simulink model "FinalRobot"  (R2021b)
settings: Solver=ode23t  StartTime=0.0  StopTime=120  MaxStep=3e-3  RelTol=1e-3
undefined symbols (not defined in the file): Amor1, Amor2, Amor3, Amor4, Amor5, B_Verin1, B_Verin2, B_Verin3, B_Verin4, B_Verin5, H_Verin1, H_Verin2, H_Verin3, H_Verin4, H_Verin5, k, K, Middle_Sensing, Sensing_1, Sensing_2, Wall_1, Wall_10, Wall_11, Wall_2, Wall_3, Wall_4, Wall_5, Wall_6, Wall_7, Wall_8, Wall_9, X, Y, Z
libraries: sm_lib x237, nesl_utility x60
(part 2 of 8)

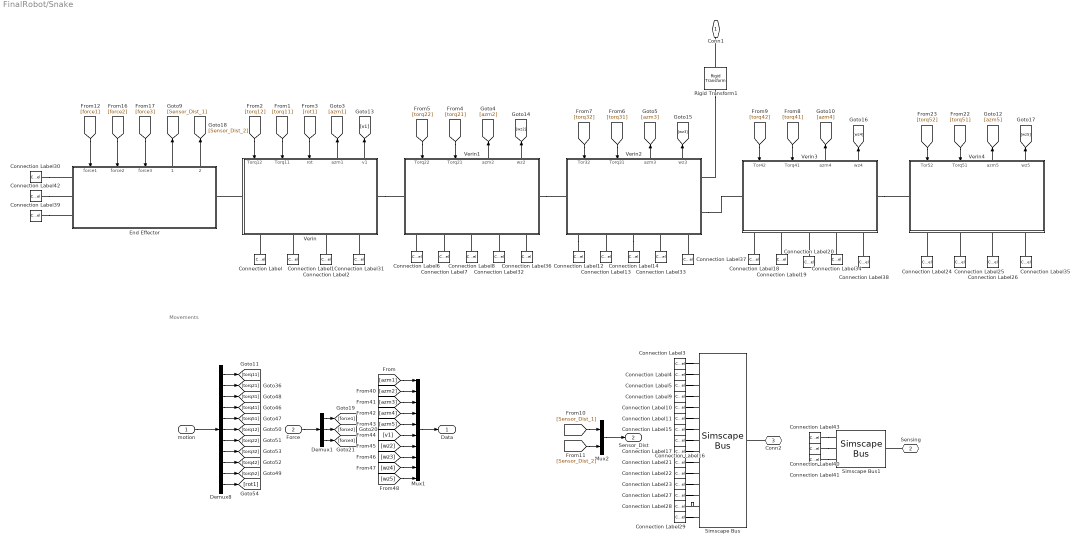
== system FinalRobot/Snake ==
  note: Movements
  motion : Inport
  Force : Inport  Port=2
  Connection Label : ConnectionLabel
  Connection Label1 : ConnectionLabel  Label=Label2
  Connection Label10 : ConnectionLabel  Label=Label5
  Connection Label11 : ConnectionLabel  Label=Label6
  Connection Label12 : ConnectionLabel  Label=Label7
  Connection Label13 : ConnectionLabel  Label=Label8
  Connection Label14 : ConnectionLabel  Label=Label9
  Connection Label15 : ConnectionLabel  Label=Label7
  Connection Label16 : ConnectionLabel  Label=Label8
  Connection Label17 : ConnectionLabel  Label=Label9
  Connection Label18 : ConnectionLabel  Label=Label10
  Connection Label19 : ConnectionLabel  Label=Label11
  Connection Label2 : ConnectionLabel  Label=Label3
  Connection Label20 : ConnectionLabel  Label=Label12
  Connection Label21 : ConnectionLabel  Label=Label10
  Connection Label22 : ConnectionLabel  Label=Label11
  Connection Label23 : ConnectionLabel  Label=Label12
  Connection Label24 : ConnectionLabel  Label=Label13
  Connection Label25 : ConnectionLabel  Label=Label14
  Connection Label26 : ConnectionLabel  Label=Label15
  Connection Label27 : ConnectionLabel  Label=Label13
  Connection Label28 : ConnectionLabel  Label=Label14
  Connection Label29 : ConnectionLabel  Label=Label15
  Connection Label3 : ConnectionLabel
  Connection Label30 : ConnectionLabel  Label=Label16
  Connection Label31 : ConnectionLabel  Label=Ref1
  Connection Label32 : ConnectionLabel  Label=Ref1
  Connection Label33 : ConnectionLabel  Label=Ref2
  Connection Label34 : ConnectionLabel  Label=Ref3
  Connection Label35 : ConnectionLabel  Label=Ref4
  Connection Label36 : ConnectionLabel  Label=Ref2
  Connection Label37 : ConnectionLabel  Label=Ref3
  Connection Label38 : ConnectionLabel  Label=Ref4
  Connection Label39 : ConnectionLabel  Label=Label17
  Connection Label4 : ConnectionLabel  Label=Label2
  Connection Label40 : ConnectionLabel  Label=Label16
  Connection Label41 : ConnectionLabel  Label=Label17
  Connection Label42 : ConnectionLabel  Label=Label18
  Connection Label43 : ConnectionLabel  Label=Label18
  Connection Label5 : ConnectionLabel  Label=Label3
  Connection Label6 : ConnectionLabel  Label=Label4
  Connection Label7 : ConnectionLabel  Label=Label5
  Connection Label8 : ConnectionLabel  Label=Label6
  Connection Label9 : ConnectionLabel  Label=Label4
  Demux1 : Demux  Outputs=3
  Demux8 : Demux  Outputs=11
  End Effector : Subsystem
      settings: PortSchema="{\"entries\":[{\"content\":{\"sides\":[{\"content\":{\"connectorIds\":[\"LConn1\",\"LConn2\",\"LConn3\"]},\"type\":\"ConnectorPlacement.EquallySpacedRectSide\",\"uuid\":\"5cdd056e-886a-4e79-8899-044af396038d\"},{\"content\":{\"connectorIds\":[\"RConn1\"],\"side\":\"RIGHT\"},\"type\":\"ConnectorPlacement.EquallySpacedRectSide\",\"uuid\":\"cf985096-d37a-46e5-b464-4af5c863f88b\"},{\"content\":{\"connectorIds\":[\"In1\",\"In2\",\"In3\",\"Out1\",\"Out2\"],\"side\":\"TOP\"},\"type\":\"ConnectorPlacement.EquallySpacedRectSide\",\"uuid\":\"be1169e8-83ff-4042-b398-0e1dc3f716bc\"}]},\"type\":\"ConnectorPlacement.EquallySpacedConnector\",\"uuid\":\"d39d92c9-4302-400d-962a-d4b186813480\"}],\"packageUris\":[\"http://schema.mathworks.com/mf0/Connector/R2020b\"],\"version\":\"1.0\"}"
      mask Display: image('$imagefile'); % Use "Edit Image" on toolstrip to change.
  Mux1 : Mux  Inputs=10
  Mux2 : Mux  Inputs=2
  Rigid Transform1 : sm_lib/Frames and Transforms/Rigid Transform  TranslationMethod=Cartesian  TranslationStandardOffset=0  TranslationLengthUnit=m  TranslationStandardAxis=+Z  TranslationCartesianOffset=[-0.1 -0.2 0.1]  TranslationROffset=0  TranslationROffsetUnits=m  TranslationZOffset=0  TranslationZOffsetUnits=m  TranslationThetaOffset=0  TranslationThetaOffsetUnits=deg  RotationMethod=StandardAxis  RotationAngleUnits=deg  RotationStandardAxis=+Z  RotationAngle=30  RotationArbitraryAxis=[0 0 1]  FollAlignAxisA=+X  BaseAlignAxisA=+Y  FollAlignAxisB=+Y  BaseAlignAxisB=+Z  RotationSequenceAxes=FollowerAxes  RotationSequence=XYX  RotationSequenceAngles=[0 0 0]  RotationSequenceAnglesUnits=deg  RotationMatrix=[1 0 0; 0 1 0; 0 0 1]
  Simscape Bus : SimscapeBus  HierarchyStrings=Amor1;H_Verin1;B_Verin1;Amor2;H_Verin2;B_Verin2;Amor3;H_Verin3;B_Verin3;Amor4;H_Verin4;B_Verin4;Amor5;H_Verin5;B_Verin5
  Simscape Bus1 : SimscapeBus  HierarchyStrings=Middle_Sensing;Sensing_1;Sensing_2
  Verin : Subsystem
      settings: PortSchema="{\"entries\":[{\"content\":{\"sides\":[{\"content\":{\"connectorIds\":[\"LConn1\"]},\"type\":\"ConnectorPlacement.EquallySpacedRectSide\",\"uuid\":\"c3246ee3-eb2d-4c48-a7f8-29eef62ed6cd\"},{\"content\":{\"connectorIds\":[\"RConn1\"],\"side\":\"RIGHT\"},\"type\":\"ConnectorPlacement.EquallySpacedRectSide\",\"uuid\":\"dd74c587-cb0d-4684-823f-ccc260fba800\"},{\"content\":{\"connectorIds\":[\"In1\",\"In2\",\"In3\",\"Out1\",\"Out2\"],\"side\":\"TOP\"},\"type\":\"ConnectorPlacement.EquallySpacedRectSide\",\"uuid\":\"65ea7381-0dcf-4a70-96d8-66f9da1f3035\"},{\"content\":{\"connectorIds\":[\"RConn2\",\"RConn3\",\"RConn4\",\"RConn5\"],\"side\":\"BOTTOM\"},\"type\":\"ConnectorPlacement.EquallySpacedRectSide\",\"uuid\":\"fb9c5bb7-17a2-4c30-b9f8-fa15cd56ac19\"}]},\"type\":\"ConnectorPlacement.EquallySpacedConnector\",\"uuid\":\"772b1dde-44da-42b0-bd8c-81ff8dd9042a\"}],\"packageUris\":[\"http://schema.mathworks.com/mf0/Connector/R2020b\"],\"version\":\"1.0\"}"
      mask Display: image('$imagefile'); % Use "Edit Image" on toolstrip to change.
  Verin1 : Subsystem
      settings: PortSchema="{\"entries\":[{\"content\":{\"sides\":[{\"content\":{\"connectorIds\":[\"LConn1\"]},\"type\":\"ConnectorPlacement.EquallySpacedRectSide\",\"uuid\":\"c3246ee3-eb2d-4c48-a7f8-29eef62ed6cd\"},{\"content\":{\"connectorIds\":[\"RConn1\"],\"side\":\"RIGHT\"},\"type\":\"ConnectorPlacement.EquallySpacedRectSide\",\"uuid\":\"dd74c587-cb0d-4684-823f-ccc260fba800\"},{\"content\":{\"connectorIds\":[\"In1\",\"In2\",\"Out1\",\"Out2\"],\"side\":\"TOP\"},\"type\":\"ConnectorPlacement.EquallySpacedRectSide\",\"uuid\":\"65ea7381-0dcf-4a70-96d8-66f9da1f3035\"},{\"content\":{\"connectorIds\":[\"RConn2\",\"RConn3\",\"RConn4\",\"RConn5\",\"RConn6\"],\"side\":\"BOTTOM\"},\"type\":\"ConnectorPlacement.EquallySpacedRectSide\",\"uuid\":\"fb9c5bb7-17a2-4c30-b9f8-fa15cd56ac19\"}]},\"type\":\"ConnectorPlacement.EquallySpacedConnector\",\"uuid\":\"772b1dde-44da-42b0-bd8c-81ff8dd9042a\"}],\"packageUris\":[\"http://schema.mathworks.com/mf0/Connector/R2020b\"],\"version\":\"1.0\"}"
      mask Display: image('$imagefile'); % Use "Edit Image" on toolstrip to change.
  Verin2 : Subsystem
      settings: PortSchema="{\"entries\":[{\"content\":{\"sides\":[{\"content\":{\"connectorIds\":[\"LConn1\"]},\"type\":\"ConnectorPlacement.EquallySpacedRectSide\",\"uuid\":\"c3246ee3-eb2d-4c48-a7f8-29eef62ed6cd\"},{\"content\":{\"connectorIds\":[\"RConn1\",\"RConn2\"],\"side\":\"RIGHT\"},\"type\":\"ConnectorPlacement.EquallySpacedRectSide\",\"uuid\":\"dd74c587-cb0d-4684-823f-ccc260fba800\"},{\"content\":{\"connectorIds\":[\"In1\",\"In2\",\"Out1\",\"Out2\"],\"side\":\"TOP\"},\"type\":\"ConnectorPlacement.EquallySpacedRectSide\",\"uuid\":\"65ea7381-0dcf-4a70-96d8-66f9da1f3035\"},{\"content\":{\"connectorIds\":[\"RConn3\",\"RConn4\",\"RConn5\",\"RConn6\",\"RConn7\"],\"side\":\"BOTTOM\"},\"type\":\"ConnectorPlacement.EquallySpacedRectSide\",\"uuid\":\"fb9c5bb7-17a2-4c30-b9f8-fa15cd56ac19\"}]},\"type\":\"ConnectorPlacement.EquallySpacedConnector\",\"uuid\":\"772b1dde-44da-42b0-bd8c-81ff8dd9042a\"}],\"packageUris\":[\"http://schema.mathworks.com/mf0/Connector/R2020b\"],\"version\":\"1.0\"}"
      mask Display: image('$imagefile'); % Use "Edit Image" on toolstrip to change.
  Verin3 : Subsystem
      settings: PortSchema="{\"entries\":[{\"content\":{\"sides\":[{\"content\":{\"connectorIds\":[\"LConn1\"]},\"type\":\"ConnectorPlacement.EquallySpacedRectSide\",\"uuid\":\"c3246ee3-eb2d-4c48-a7f8-29eef62ed6cd\"},{\"content\":{\"connectorIds\":[\"RConn1\"],\"side\":\"RIGHT\"},\"type\":\"ConnectorPlacement.EquallySpacedRectSide\",\"uuid\":\"dd74c587-cb0d-4684-823f-ccc260fba800\"},{\"content\":{\"connectorIds\":[\"In1\",\"In2\",\"Out1\",\"Out2\"],\"side\":\"TOP\"},\"type\":\"ConnectorPlacement.EquallySpacedRectSide\",\"uuid\":\"65ea7381-0dcf-4a70-96d8-66f9da1f3035\"},{\"content\":{\"connectorIds\":[\"RConn2\",\"RConn3\",\"RConn4\",\"RConn5\",\"RConn6\"],\"side\":\"BOTTOM\"},\"type\":\"ConnectorPlacement.EquallySpacedRectSide\",\"uuid\":\"fb9c5bb7-17a2-4c30-b9f8-fa15cd56ac19\"}]},\"type\":\"ConnectorPlacement.EquallySpacedConnector\",\"uuid\":\"772b1dde-44da-42b0-bd8c-81ff8dd9042a\"}],\"packageUris\":[\"http://schema.mathworks.com/mf0/Connector/R2020b\"],\"version\":\"1.0\"}"
      mask Display: image('$imagefile'); % Use "Edit Image" on toolstrip to change.
  Verin4 : Subsystem
      settings: PortSchema="{\"entries\":[{\"content\":{\"sides\":[{\"content\":{\"connectorIds\":[\"LConn1\"]},\"type\":\"ConnectorPlacement.EquallySpacedRectSide\",\"uuid\":\"c3246ee3-eb2d-4c48-a7f8-29eef62ed6cd\"},{\"content\":{\"connectorIds\":[],\"side\":\"RIGHT\"},\"type\":\"ConnectorPlacement.EquallySpacedRectSide\",\"uuid\":\"dd74c587-cb0d-4684-823f-ccc260fba800\"},{\"content\":{\"connectorIds\":[\"In1\",\"In2\",\"Out1\",\"Out2\"],\"side\":\"TOP\"},\"type\":\"ConnectorPlacement.EquallySpacedRectSide\",\"uuid\":\"65ea7381-0dcf-4a70-96d8-66f9da1f3035\"},{\"content\":{\"connectorIds\":[\"RConn1\",\"RConn2\",\"RConn3\",\"RConn4\"],\"side\":\"BOTTOM\"},\"type\":\"ConnectorPlacement.EquallySpacedRectSide\",\"uuid\":\"fb9c5bb7-17a2-4c30-b9f8-fa15cd56ac19\"}]},\"type\":\"ConnectorPlacement.EquallySpacedConnector\",\"uuid\":\"772b1dde-44da-42b0-bd8c-81ff8dd9042a\"}],\"packageUris\":[\"http://schema.mathworks.com/mf0/Connector/R2020b\"],\"version\":\"1.0\"}"
      mask Display: image('$imagefile'); % Use "Edit Image" on toolstrip to change.
  Conn1 : PMIOPort  Side=Left
  Sensing : PMIOPort  Port=2  Side=Right
  Conn2 : PMIOPort  Port=3  Side=Right
  Data : Outport
  Sensor_Dist : Outport  Port=2
  wires:
  [torq41] -> Verin3/2(Torq41)
  [torq22] -> Verin1/1(Torq22)
  [torq52] -> Verin4/1(Tor52)
  Demux8/2 -> [torq21]
  Demux8/6 -> [torq12]
  Demux8/11 -> [rot1]
  [torq11] -> Verin/2(Torq11)
  [rot1] -> Verin/3(rot)
  [torq21] -> Verin1/2(Torq21)
  [torq51] -> Verin4/2(Torq51)
  [torq42] -> Verin3/1(Tor42)
  Demux8/9 -> [torq42]
  Demux8/7 -> [torq22]
  [torq32] -> Verin2/1(Tor32)
  Demux8/3 -> [torq31]
  Demux8/4 -> [torq41]
  [torq31] -> Verin2/2(Torq31)
  [torq12] -> Verin/1(Torq12)
  Demux8/10 -> [torq52]
  Demux8/5 -> [torq51]
  Demux8/1 -> [torq11]
  Demux8/8 -> [torq32]
  motion/1 -> Demux8/1
  Mux1/1 -> Data/1
  [azm1] -> Mux1/1
  Verin/1(azm1) -> [azm1]
  Verin1/1(azm2) -> [azm2]
  Verin2/1(azm3) -> [azm3]
  Verin3/1(azm4) -> [azm4]
  Verin4/1(azm5) -> [azm5]
  [azm2] -> Mux1/2
  [azm3] -> Mux1/3
  [azm4] -> Mux1/4
  [azm5] -> Mux1/5
  Verin/2(v1) -> [v1]
  Verin1/2(wz2) -> [wz2]
  Verin2/2(wz3) -> [wz3]
  Verin3/2(wz4) -> [wz4]
  Verin4/2(wz5) -> [wz5]
  [wz3] -> Mux1/8
  [wz2] -> Mux1/7
  [v1] -> Mux1/6
  [wz4] -> Mux1/9
  [wz5] -> Mux1/10
  End Effector/1(Sensor_Dist_1) -> [Sensor_Dist_1]
  End Effector/2(Sensor_Dist_2) -> [Sensor_Dist_2]
  [Sensor_Dist_1] -> Mux2/1
  [Sensor_Dist_2] -> Mux2/2
  Mux2/1 -> Sensor_Dist/1
  Force/1 -> Demux1/1
  Demux1/1 -> [force1]
  Demux1/2 -> [force2]
  Demux1/3 -> [force3]
  [force2] -> End Effector/2(force2)
  [force1] -> End Effector/1(force1)
  [force3] -> End Effector/3(force3)
  connections:
  Verin2/RConn2 -- Verin3/LConn1
  Verin3/RConn1 -- Verin4/LConn1
  Verin1/RConn1 -- Verin2/LConn1
  Rigid Transform1/LConn1 -- Conn1/RConn1
  Conn2/RConn1 -- Simscape Bus/RConn1
  Connection Label/LConn1 -- Verin/RConn2
  Connection Label1/LConn1 -- Verin/RConn3
  Connection Label2/LConn1 -- Verin/RConn4
  Connection Label5/LConn1 -- Simscape Bus/LConn3
  Connection Label3/LConn1 -- Simscape Bus/LConn1
  Connection Label4/LConn1 -- Simscape Bus/LConn2
  Connection Label6/LConn1 -- Verin1/RConn2
  Connection Label7/LConn1 -- Verin1/RConn3
  Connection Label8/LConn1 -- Verin1/RConn4
  Connection Label9/LConn1 -- Simscape Bus/LConn4
  Connection Label10/LConn1 -- Simscape Bus/LConn5
  Connection Label11/LConn1 -- Simscape Bus/LConn6
  Verin2/RConn5 -- Connection Label14/LConn1
  Connection Label13/LConn1 -- Verin2/RConn4
  Verin2/RConn3 -- Connection Label12/LConn1
  Connection Label19/LConn1 -- Verin3/RConn3
  Connection Label18/LConn1 -- Verin3/RConn2
  Connection Label20/LConn1 -- Verin3/RConn4
  Connection Label23/LConn1 -- Simscape Bus/LConn12
  Connection Label21/LConn1 -- Simscape Bus/LConn10
  Connection Label22/LConn1 -- Simscape Bus/LConn11
  Connection Label15/LConn1 -- Simscape Bus/LConn7
  Connection Label16/LConn1 -- Simscape Bus/LConn8
  Connection Label17/LConn1 -- Simscape Bus/LConn9
  Connection Label24/LConn1 -- Verin4/RConn1
  Connection Label25/LConn1 -- Verin4/RConn2
  Connection Label26/LConn1 -- Verin4/RConn3
  Connection Label27/LConn1 -- Simscape Bus/LConn13
  Connection Label29/LConn1 -- Simscape Bus/LConn15
  Simscape Bus/LConn14 -- Connection Label28/LConn1
  Connection Label31/LConn1 -- Verin/RConn5
  Connection Label32/LConn1 -- Verin1/RConn5
  Connection Label33/LConn1 -- Verin2/RConn6
  Connection Label34/LConn1 -- Verin3/RConn5
  Connection Label35/LConn1 -- Verin4/RConn4
  Connection Label36/LConn1 -- Verin1/RConn6
  Connection Label37/LConn1 -- Verin2/RConn7
  Connection Label38/LConn1 -- Verin3/RConn6
  Rigid Transform1/RConn1 -- Verin2/RConn1
  Sensing/RConn1 -- Simscape Bus1/RConn1
  Connection Label41/LConn1 -- Simscape Bus1/LConn3
  Connection Label40/LConn1 -- Simscape Bus1/LConn2
  Connection Label43/LConn1 -- Simscape Bus1/LConn1
  Connection Label30/LConn1 -- End Effector/LConn1
  Connection Label42/LConn1 -- End Effector/LConn2
  Verin/LConn1 -- End Effector/RConn1
  Connection Label39/LConn1 -- End Effector/LConn3
  Verin/RConn1 -- Verin1/LConn1

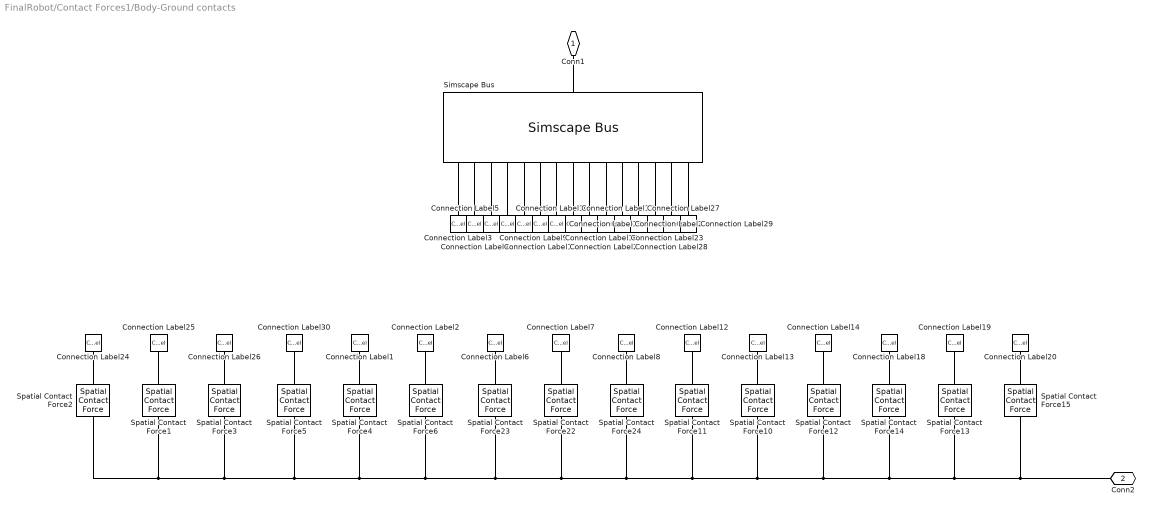
== system FinalRobot/Contact Forces1/Body-Ground contacts ==
  Connection Label1 : ConnectionLabel  Label=Label5
  Connection Label10 : ConnectionLabel  Label=Label5
  Connection Label11 : ConnectionLabel  Label=Label6
  Connection Label12 : ConnectionLabel  Label=Label10
  Connection Label13 : ConnectionLabel  Label=Label11
  Connection Label14 : ConnectionLabel  Label=Label12
  Connection Label15 : ConnectionLabel  Label=Label7
  Connection Label16 : ConnectionLabel  Label=Label8
  Connection Label17 : ConnectionLabel  Label=Label9
  Connection Label18 : ConnectionLabel  Label=Label13
  Connection Label19 : ConnectionLabel  Label=Label14
  Connection Label2 : ConnectionLabel  Label=Label6
  Connection Label20 : ConnectionLabel  Label=Label15
  Connection Label21 : ConnectionLabel  Label=Label10
  Connection Label22 : ConnectionLabel  Label=Label11
  Connection Label23 : ConnectionLabel  Label=Label12
  Connection Label24 : ConnectionLabel
  Connection Label25 : ConnectionLabel  Label=Label2
  Connection Label26 : ConnectionLabel  Label=Label3
  Connection Label27 : ConnectionLabel  Label=Label13
  Connection Label28 : ConnectionLabel  Label=Label14
  Connection Label29 : ConnectionLabel  Label=Label15
  Connection Label3 : ConnectionLabel
  Connection Label30 : ConnectionLabel  Label=Label4
  Connection Label4 : ConnectionLabel  Label=Label2
  Connection Label5 : ConnectionLabel  Label=Label3
  Connection Label6 : ConnectionLabel  Label=Label7
  Connection Label7 : ConnectionLabel  Label=Label8
  Connection Label8 : ConnectionLabel  Label=Label9
  Connection Label9 : ConnectionLabel  Label=Label4
  Simscape Bus : SimscapeBus  HierarchyStrings=Amor1;H_Verin1;B_Verin1;Amor2;H_Verin2;B_Verin2;Amor3;H_Verin3;B_Verin3;Amor4;H_Verin4;B_Verin4;Amor5;H_Verin5;B_Verin5
  Spatial Contact Force{1,3..4,6,10,12..13,15,22,24} (10 alike) : sm_lib/Forces and Torques/Spatial Contact Force  CoefficientOfDynamicFriction=Dynamic_Friction_Verin  CoefficientOfStaticFriction=Static_Friction_Verin  SenseContactBaseRotation=off  SenseContactBaseTranslation=off  NormalDamping=1e3  NormalDampingUnits=N/(m/s)  SenseContactFollowerRotation=off  SenseContactFollowerTranslation=off  SenseContactSignal=off  NormalStiffness=1e6  NormalStiffnessUnits=N/m  FrictionalCriticalVelocity=1e-3  FrictionalCriticalVelocityUnits=m/s  ZeroCrossDetectContactStartAndEnd=off  FrictionType=SmoothStickSlip  SenseFrictionalForceMagnitude=off  SenseNormalForceMagnitude=off  NormalForceType=SmoothSpringDamper  SenseNormalVelocity=off  SenseSeparationDistance=off  SenseTangentialVelocity=off  SenseTangentialVelocityMagnitude=off  NormalTransitionRegionWidth=1e-4  NormalTransitionRegionWidthUnits=m
  Spatial Contact Force{2,5,11,14,23} (5 alike) : sm_lib/Forces and Torques/Spatial Contact Force  CoefficientOfDynamicFriction=Dynamic_Friction_Amor  CoefficientOfStaticFriction=Static_Friction_Amor  SenseContactBaseRotation=off  SenseContactBaseTranslation=off  NormalDamping=1e3  NormalDampingUnits=N/(m/s)  SenseContactFollowerRotation=off  SenseContactFollowerTranslation=off  SenseContactSignal=off  NormalStiffness=1e6  NormalStiffnessUnits=N/m  FrictionalCriticalVelocity=1e-3  FrictionalCriticalVelocityUnits=m/s  ZeroCrossDetectContactStartAndEnd=off  FrictionType=SmoothStickSlip  SenseFrictionalForceMagnitude=off  SenseNormalForceMagnitude=off  NormalForceType=SmoothSpringDamper  SenseNormalVelocity=off  SenseSeparationDistance=off  SenseTangentialVelocity=off  SenseTangentialVelocityMagnitude=off  NormalTransitionRegionWidth=1e-4  NormalTransitionRegionWidthUnits=m
  Conn1 : PMIOPort  Side=Left
  Conn2 : PMIOPort  Port=2  Side=Right
  connections:
  Connection Label15/LConn1 -- Simscape Bus/LConn7
  Spatial Contact Force2/LConn1 -- Spatial Contact Force1/LConn1 -- Spatial Contact Force3/LConn1 -- Spatial Contact Force5/LConn1 -- Spatial Contact Force4/LConn1 -- Spatial Contact Force6/LConn1 -- Spatial Contact Force23/LConn1 -- Spatial Contact Force22/LConn1 -- Spatial Contact Force24/LConn1 -- Spatial Contact Force11/LConn1 -- Spatial Contact Force10/LConn1 -- Spatial Contact Force12/LConn1 -- Conn2/RConn1 -- Spatial Contact Force15/LConn1 -- Spatial Contact Force13/LConn1 -- Spatial Contact Force14/LConn1
  Connection Label26/LConn1 -- Spatial Contact Force3/RConn1
  Connection Label30/LConn1 -- Spatial Contact Force5/RConn1
  Connection Label24/LConn1 -- Spatial Contact Force2/RConn1
  Connection Label27/LConn1 -- Simscape Bus/LConn13
  Connection Label29/LConn1 -- Simscape Bus/LConn15
  Connection Label18/LConn1 -- Spatial Contact Force14/RConn1
  Connection Label14/LConn1 -- Spatial Contact Force12/RConn1
  Connection Label20/LConn1 -- Spatial Contact Force15/RConn1
  Connection Label11/LConn1 -- Simscape Bus/LConn6
  Connection Label1/LConn1 -- Spatial Contact Force4/RConn1
  Connection Label8/LConn1 -- Spatial Contact Force24/RConn1
  Connection Label13/LConn1 -- Spatial Contact Force10/RConn1
  Simscape Bus/LConn14 -- Connection Label28/LConn1
  Connection Label25/LConn1 -- Spatial Contact Force1/RConn1
  Connection Label7/LConn1 -- Spatial Contact Force22/RConn1
  Connection Label10/LConn1 -- Simscape Bus/LConn5
  Connection Label16/LConn1 -- Simscape Bus/LConn8
  Connection Label22/LConn1 -- Simscape Bus/LConn11
  Connection Label3/LConn1 -- Simscape Bus/LConn1
  Connection Label17/LConn1 -- Simscape Bus/LConn9
  Connection Label23/LConn1 -- Simscape Bus/LConn12
  Connection Label6/LConn1 -- Spatial Contact Force23/RConn1
  Connection Label4/LConn1 -- Simscape Bus/LConn2
  Connection Label5/LConn1 -- Simscape Bus/LConn3
  Connection Label2/LConn1 -- Spatial Contact Force6/RConn1
  Connection Label12/LConn1 -- Spatial Contact Force11/RConn1
  Connection Label19/LConn1 -- Spatial Contact Force13/RConn1
  Connection Label9/LConn1 -- Simscape Bus/LConn4
  Connection Label21/LConn1 -- Simscape Bus/LConn10
  Conn1/RConn1 -- Simscape Bus/RConn1

== system FinalRobot/Contact Forces1/Subsystem3 ==
  Simscape Bus1 : SimscapeBus  HierarchyStrings=Middle_Sensing;Sensing_1;Sensing_2
  Simscape Bus2 : SimscapeBus  HierarchyStrings=Wall_1;Wall_2;Wall_3;Wall_4;Wall_5;Wall_6;Wall_7;Wall_8;Wall_9;Wall_10;Wall_11
  Subsystem : Subsystem
      settings: PortSchema="{\"entries\":[{\"content\":{\"sides\":[{\"content\":{\"connectorIds\":[]},\"type\":\"ConnectorPlacement.EquallySpacedRectSide\",\"uuid\":\"68d41a2c-cf4f-4266-9bb2-d19176523fa8\"},{\"content\":{\"connectorIds\":[],\"side\":\"RIGHT\"},\"type\":\"ConnectorPlacement.EquallySpacedRectSide\",\"uuid\":\"fed068d2-51f7-41d7-8fa2-5f11aa30b23c\"},{\"content\":{\"connectorIds\":[\"LConn1\",\"Out1\"],\"side\":\"TOP\"},\"type\":\"ConnectorPlacement.EquallySpacedRectSide\",\"uuid\":\"b5637d28-03b4-4ccb-b57f-dccf0e87748a\"},{\"content\":{\"connectorIds\":[\"RConn1\",\"RConn2\",\"RConn3\",\"RConn4\",\"RConn5\",\"RConn6\",\"RConn7\",\"RConn8\",\"RConn9\",\"RConn10\",\"RConn11\"],\"side\":\"BOTTOM\"},\"type\":\"ConnectorPlacement.EquallySpacedRectSide\",\"uuid\":\"554c0383-4a72-43a1-a6a1-ce5953181375\"}]},\"type\":\"ConnectorPlacement.EquallySpacedConnector\",\"uuid\":\"ce1fbdf9-62dc-494f-9c60-f0c11efaa8b9\"}],\"packageUris\":[\"http://schema.mathworks.com/mf0/Connector/R2020b\"],\"version\":\"1.0\"}"
  Subsystem1 : Subsystem
      settings: PortSchema="{\"entries\":[{\"content\":{\"sides\":[{\"content\":{\"connectorIds\":[]},\"type\":\"ConnectorPlacement.EquallySpacedRectSide\",\"uuid\":\"68d41a2c-cf4f-4266-9bb2-d19176523fa8\"},{\"content\":{\"connectorIds\":[],\"side\":\"RIGHT\"},\"type\":\"ConnectorPlacement.EquallySpacedRectSide\",\"uuid\":\"fed068d2-51f7-41d7-8fa2-5f11aa30b23c\"},{\"content\":{\"connectorIds\":[\"LConn1\",\"Out1\"],\"side\":\"TOP\"},\"type\":\"ConnectorPlacement.EquallySpacedRectSide\",\"uuid\":\"b5637d28-03b4-4ccb-b57f-dccf0e87748a\"},{\"content\":{\"connectorIds\":[\"RConn1\",\"RConn2\",\"RConn3\",\"RConn4\",\"RConn5\",\"RConn6\",\"RConn7\",\"RConn8\",\"RConn9\",\"RConn10\",\"RConn11\"],\"side\":\"BOTTOM\"},\"type\":\"ConnectorPlacement.EquallySpacedRectSide\",\"uuid\":\"554c0383-4a72-43a1-a6a1-ce5953181375\"}]},\"type\":\"ConnectorPlacement.EquallySpacedConnector\",\"uuid\":\"ce1fbdf9-62dc-494f-9c60-f0c11efaa8b9\"}],\"packageUris\":[\"http://schema.mathworks.com/mf0/Connector/R2020b\"],\"version\":\"1.0\"}"
  Subsystem2 : Subsystem
      settings: PortSchema="{\"entries\":[{\"content\":{\"sides\":[{\"content\":{\"connectorIds\":[]},\"type\":\"ConnectorPlacement.EquallySpacedRectSide\",\"uuid\":\"68d41a2c-cf4f-4266-9bb2-d19176523fa8\"},{\"content\":{\"connectorIds\":[],\"side\":\"RIGHT\"},\"type\":\"ConnectorPlacement.EquallySpacedRectSide\",\"uuid\":\"fed068d2-51f7-41d7-8fa2-5f11aa30b23c\"},{\"content\":{\"connectorIds\":[\"LConn1\",\"Out1\"],\"side\":\"TOP\"},\"type\":\"ConnectorPlacement.EquallySpacedRectSide\",\"uuid\":\"b5637d28-03b4-4ccb-b57f-dccf0e87748a\"},{\"content\":{\"connectorIds\":[\"RConn1\",\"RConn2\",\"RConn3\",\"RConn4\",\"RConn5\",\"RConn6\",\"RConn7\",\"RConn8\",\"RConn9\",\"RConn10\",\"RConn11\"],\"side\":\"BOTTOM\"},\"type\":\"ConnectorPlacement.EquallySpacedRectSide\",\"uuid\":\"554c0383-4a72-43a1-a6a1-ce5953181375\"}]},\"type\":\"ConnectorPlacement.EquallySpacedConnector\",\"uuid\":\"ce1fbdf9-62dc-494f-9c60-f0c11efaa8b9\"}],\"packageUris\":[\"http://schema.mathworks.com/mf0/Connector/R2020b\"],\"version\":\"1.0\"}"
  Conn1 : PMIOPort  Side=Left
  Conn2 : PMIOPort  Port=2  Side=Right
  Contact2 : Outport
  Contact1 : Outport  Port=2
  Middle_Contact : Outport  Port=3
  wires:
  Subsystem2/1(Middle_Contact) -> Middle_Contact/1
  Subsystem1/1(Contact1) -> Contact1/1
  Subsystem/1(Contact2) -> Contact2/1
  connections:
  Simscape Bus2/LConn9 -- Subsystem/RConn9 -- Subsystem1/RConn9 -- Subsystem2/RConn9
  Simscape Bus2/LConn11 -- Subsystem2/RConn11 -- Subsystem1/RConn11 -- Subsystem/RConn11
  Simscape Bus2/LConn3 -- Subsystem/RConn3 -- Subsystem1/RConn3 -- Subsystem2/RConn3
  Simscape Bus2/LConn10 -- Subsystem/RConn10 -- Subsystem2/RConn10 -- Subsystem1/RConn10
  Simscape Bus2/LConn4 -- Subsystem1/RConn4 -- Subsystem2/RConn4 -- Subsystem/RConn4
  Simscape Bus2/LConn1 -- Subsystem/RConn1 -- Subsystem1/RConn1 -- Subsystem2/RConn1
  Simscape Bus1/LConn1 -- Subsystem2/LConn1
  Simscape Bus2/LConn6 -- Subsystem/RConn6 -- Subsystem1/RConn6 -- Subsystem2/RConn6
  Simscape Bus2/LConn5 -- Subsystem/RConn5 -- Subsystem1/RConn5 -- Subsystem2/RConn5
  Simscape Bus2/LConn8 -- Subsystem/RConn8 -- Subsystem1/RConn8 -- Subsystem2/RConn8
  Simscape Bus2/LConn7 -- Subsystem/RConn7 -- Subsystem2/RConn7 -- Subsystem1/RConn7
  Simscape Bus2/LConn2 -- Subsystem/RConn2 -- Subsystem1/RConn2 -- Subsystem2/RConn2
  Simscape Bus1/LConn2 -- Subsystem1/LConn1
  Simscape Bus1/LConn3 -- Subsystem/LConn1
  Simscape Bus2/RConn1 -- Conn2/RConn1
  Simscape Bus1/RConn1 -- Conn1/RConn1

== system FinalRobot/Snake/End Effector ==
  force1 : Inport
  force2 : Inport  Port=2
  force3 : Inport  Port=3
  Brick Solid1 : sm_lib/Body Elements/Brick Solid  GraphicAmbientColor=[0.15 0.15 0.15 1.0]  BasedOnType=Density  BrickDimensions=[1.5 0.7 0.7]*5  BrickDimensionUnits=cm  CenterOfMass=[0 0 0]  CenterOfMassUnits=m  GraphicDiffuseColor=[0.9411765 0.9411765 0.9411765]  Density=1000  DensityUnits=kg/m^3  DoExposeReferenceFrame=on  GraphicEmissiveColor=[0.0 0.0 0.0 1.0]  ExportEntireGeometry=off  SerializedFrames=<Frames><Frame><Id>Frame1</Id><Value><Name>F1</Name><Origin><Source>GeometricFeature</Source><FeatureName>-x surface</FeatureName></Origin><PrimaryAxis><DefinedDirection>+Z</DefinedDirection><Source>ReferenceFrame</Source><SourceDirection>+Z</SourceDirection><FeatureName></FeatureName></PrimaryAxis><SecondaryAxis><DefinedDirection>+X</DefinedDirection><Source>ReferenceFrame</Source><SourceDirection>+X</SourceDirection><FeatureName></FeatureName></SecondaryAxis></Value></Frame></Frames>  MarkerShape=Sphere  MarkerSize=10  GraphicType=FromGeometry  InertiaType=CalculateFromGeometry  Mass=1  MassUnits=kg  MomentsOfInertia=[1 1 1]  MomentsOfInertiaUnits=kg*m^2  GraphicOpacity=1.0  ProductsOfInertia=[0 0 0]  ProductsOfInertiaUnits=kg*m^2  GraphicShininess=75  GraphicSpecularColor=[0.5 0.5 0.5 1.0]  GraphicVisPropType=SimpleVisualProperties
  Middle_Sensor : sm_lib/Body Elements/Spherical Solid  GraphicAmbientColor=[0.15 0.15 0.15 1.0]  BasedOnType=Density  CenterOfMass=[0 0 0]  CenterOfMassUnits=m  GraphicDiffuseColor=[0.9411765 0.9411765 0.9411765]  Density=1000  DensityUnits=kg/m^3  DoExposeReferenceFrame=on  GraphicEmissiveColor=[0.0 0.0 0.0 1.0]  ExportEntireGeometry=on  SerializedExposedGeometries=<ExposedGeometries><ExposedGeometry><RawGeometryId>entire</RawGeometryId><ExposedGeometryId>G</ExposedGeometryId></ExposedGeometry></ExposedGeometries>  SerializedFrames=<Frames/>  MarkerShape=Sphere  MarkerSize=10  GraphicType=FromGeometry  InertiaType=CalculateFromGeometry  Mass=1  MassUnits=kg  MomentsOfInertia=[1 1 1]  MomentsOfInertiaUnits=kg*m^2  GraphicOpacity=1.0  ProductsOfInertia=[0 0 0]  ProductsOfInertiaUnits=kg*m^2  GraphicShininess=75  GraphicSpecularColor=[0.5 0.5 0.5 1.0]  SphereRadius=0.1  SphereRadiusUnits=cm  GraphicVisPropType=SimpleVisualProperties
  PS-Simulink Converter : nesl_utility/PS-Simulink Converter  PhysicalDomain=network_engine_domain  SubClassName=ps_output  LeftPortType=input  RightPortType=output  PseudoPeriodic=off  Frequencies=[]  Unit=inherit  AffineConversion=off
      settings: SourceProductBaseCode=PW,SS
  PS-Simulink Converter1 : nesl_utility/PS-Simulink Converter  PhysicalDomain=network_engine_domain  SubClassName=ps_output  LeftPortType=input  RightPortType=output  PseudoPeriodic=off  Frequencies=[]  Unit=inherit  AffineConversion=off
      settings: SourceProductBaseCode=PW,SS
  Prismatic Joint : sm_lib/Joints/Prismatic Joint  JointMode=Normal  SenseConstraintForce=off  SenseConstraintForceX=off  SenseConstraintForceY=off  SenseConstraintForceZ=off  SenseConstraintTorque=off  SenseConstraintTorqueX=off  SenseConstraintTorqueY=off  SenseConstraintTorqueZ=off  SenseTotalForce=off  SenseTotalForceX=off  SenseTotalForceY=off  SenseTotalForceZ=off  SenseTotalTorque=off  SenseTotalTorqueX=off  SenseTotalTorqueY=off  SenseTotalTorqueZ=off  CompositeWrenchDir=FollowerOnBase  CompositeWrenchFrame=BaseFrame  EquilibriumPosition=0.1  EquilibriumPositionUnits=m  SpringStiffness=6.8e-3  SpringStiffnessUnits=N/m  DampingCoefficient=6.8e-4  DampingCoefficientUnits=N/(m/s)  TorqueActuationMode=InputTorque  MotionActuationMode=ComputedMotion  SensePosition=off  SenseVelocity=off  SenseAcceleration=off  SenseTorqueForce=off  SenseLowerLimitTorqueForce=off  SenseUpperLimitTorqueForce=off  LowerLimitSpecify=on  LowerLimitBound=0.1  LowerLimitBoundUnits=m  LowerLimitStiffness=1e6  LowerLimitStiffnessUnits=N/m  LowerLimitDamping=1e3  LowerLimitDampingUnits=N/(m/s)  LowerLimitTransitionRegionWidth=1e-4  LowerLimitTransitionRegionWidthUnits=m  UpperLimitSpecify=off  UpperLimitBound=1  UpperLimitBoundUnits=m  UpperLimitStiffness=1e6  UpperLimitStiffnessUnits=N/m  UpperLimitDamping=1e3  UpperLimitDampingUnits=N/(m/s)  UpperLimitTransitionRegionWidth=1e-4  UpperLimitTransitionRegionWidthUnits=m  PositionTargetSpecify=on  PositionTargetPriority=High  PositionTargetValue=0.1  PositionTargetValueUnits=m  VelocityTargetSpecify=off  VelocityTargetPriority=High  VelocityTargetValue=0  VelocityTargetValueUnits=m/s
  Prismatic Joint1 : sm_lib/Joints/Prismatic Joint  JointMode=Normal  SenseConstraintForce=off  SenseConstraintForceX=off  SenseConstraintForceY=off  SenseConstraintForceZ=off  SenseConstraintTorque=off  SenseConstraintTorqueX=off  SenseConstraintTorqueY=off  SenseConstraintTorqueZ=off  SenseTotalForce=off  SenseTotalForceX=off  SenseTotalForceY=off  SenseTotalForceZ=off  SenseTotalTorque=off  SenseTotalTorqueX=off  SenseTotalTorqueY=off  SenseTotalTorqueZ=off  CompositeWrenchDir=FollowerOnBase  CompositeWrenchFrame=BaseFrame  EquilibriumPosition=0  EquilibriumPositionUnits=m  SpringStiffness=6.8e-3  SpringStiffnessUnits=N/m  DampingCoefficient=6.8e-4  DampingCoefficientUnits=N/(m/s)  TorqueActuationMode=InputTorque  MotionActuationMode=ComputedMotion  SensePosition=off  SenseVelocity=off  SenseAcceleration=off  SenseTorqueForce=off  SenseLowerLimitTorqueForce=off  SenseUpperLimitTorqueForce=off  LowerLimitSpecify=off  LowerLimitBound=-1  LowerLimitBoundUnits=m  LowerLimitStiffness=1e6  LowerLimitStiffnessUnits=N/m  LowerLimitDamping=1e3  LowerLimitDampingUnits=N/(m/s)  LowerLimitTransitionRegionWidth=1e-4  LowerLimitTransitionRegionWidthUnits=m  UpperLimitSpecify=off  UpperLimitBound=1  UpperLimitBoundUnits=m  UpperLimitStiffness=1e6  UpperLimitStiffnessUnits=N/m  UpperLimitDamping=1e3  UpperLimitDampingUnits=N/(m/s)  UpperLimitTransitionRegionWidth=1e-4  UpperLimitTransitionRegionWidthUnits=m  PositionTargetSpecify=off  PositionTargetPriority=High  PositionTargetValue=0  PositionTargetValueUnits=m  VelocityTargetSpecify=off  VelocityTargetPriority=High  VelocityTargetValue=0  VelocityTargetValueUnits=m/s
  Prismatic Joint3 : sm_lib/Joints/Prismatic Joint  JointMode=Normal  SenseConstraintForce=off  SenseConstraintForceX=off  SenseConstraintForceY=off  SenseConstraintForceZ=off  SenseConstraintTorque=off  SenseConstraintTorqueX=off  SenseConstraintTorqueY=off  SenseConstraintTorqueZ=off  SenseTotalForce=off  SenseTotalForceX=off  SenseTotalForceY=off  SenseTotalForceZ=off  SenseTotalTorque=off  SenseTotalTorqueX=off  SenseTotalTorqueY=off  SenseTotalTorqueZ=off  CompositeWrenchDir=FollowerOnBase  CompositeWrenchFrame=BaseFrame  EquilibriumPosition=0.1  EquilibriumPositionUnits=m  SpringStiffness=6.8e-3  SpringStiffnessUnits=N/m  DampingCoefficient=6.8e-4  DampingCoefficientUnits=N/(m/s)  TorqueActuationMode=InputTorque  MotionActuationMode=ComputedMotion  SensePosition=off  SenseVelocity=off  SenseAcceleration=off  SenseTorqueForce=off  SenseLowerLimitTorqueForce=off  SenseUpperLimitTorqueForce=off  LowerLimitSpecify=on  LowerLimitBound=0.1  LowerLimitBoundUnits=m  LowerLimitStiffness=1e6  LowerLimitStiffnessUnits=N/m  LowerLimitDamping=1e3  LowerLimitDampingUnits=N/(m/s)  LowerLimitTransitionRegionWidth=1e-4  LowerLimitTransitionRegionWidthUnits=m  UpperLimitSpecify=off  UpperLimitBound=1  UpperLimitBoundUnits=m  UpperLimitStiffness=1e6  UpperLimitStiffnessUnits=N/m  UpperLimitDamping=1e3  UpperLimitDampingUnits=N/(m/s)  UpperLimitTransitionRegionWidth=1e-4  UpperLimitTransitionRegionWidthUnits=m  PositionTargetSpecify=on  PositionTargetPriority=High  PositionTargetValue=0.1  PositionTargetValueUnits=m  VelocityTargetSpecify=off  VelocityTargetPriority=High  VelocityTargetValue=0  VelocityTargetValueUnits=m/s
  Rigid Transform : sm_lib/Frames and Transforms/Rigid Transform  TranslationMethod=None  TranslationStandardOffset=8  TranslationLengthUnit=cm  TranslationStandardAxis=+Z  TranslationCartesianOffset=[0 -60 0]  TranslationROffset=0  TranslationROffsetUnits=m  TranslationZOffset=0  TranslationZOffsetUnits=m  TranslationThetaOffset=0  TranslationThetaOffsetUnits=deg  RotationMethod=StandardAxis  RotationAngleUnits=deg  RotationStandardAxis=+X  RotationAngle=90  RotationArbitraryAxis=[0 0 1]  FollAlignAxisA=+X  BaseAlignAxisA=+Y  FollAlignAxisB=+Y  BaseAlignAxisB=+Z  RotationSequenceAxes=FollowerAxes  RotationSequence=XYX  RotationSequenceAngles=[0 0 0]  RotationSequenceAnglesUnits=deg  RotationMatrix=[1 0 0; 0 1 0; 0 0 1]
  Rigid Transform1 : sm_lib/Frames and Transforms/Rigid Transform  TranslationMethod=None  TranslationStandardOffset=8  TranslationLengthUnit=cm  TranslationStandardAxis=+Z  TranslationCartesianOffset=[0 60 0]  TranslationROffset=0  TranslationROffsetUnits=m  TranslationZOffset=0  TranslationZOffsetUnits=m  TranslationThetaOffset=0  TranslationThetaOffsetUnits=deg  RotationMethod=StandardAxis  RotationAngleUnits=deg  RotationStandardAxis=+X  RotationAngle=-90  RotationArbitraryAxis=[0 0 1]  FollAlignAxisA=+X  BaseAlignAxisA=+Y  FollAlignAxisB=+Y  BaseAlignAxisB=+Z  RotationSequenceAxes=FollowerAxes  RotationSequence=XYX  RotationSequenceAngles=[0 0 0]  RotationSequenceAnglesUnits=deg  RotationMatrix=[1 0 0; 0 1 0; 0 0 1]
  Rigid Transform3 : sm_lib/Frames and Transforms/Rigid Transform  TranslationMethod=Cartesian  TranslationStandardOffset=8  TranslationLengthUnit=cm  TranslationStandardAxis=+Z  TranslationCartesianOffset=[20 0 0]  TranslationROffset=0  TranslationROffsetUnits=m  TranslationZOffset=0  TranslationZOffsetUnits=m  TranslationThetaOffset=0  TranslationThetaOffsetUnits=deg  RotationMethod=StandardAxis  RotationAngleUnits=deg  RotationStandardAxis=+Y  RotationAngle=-90  RotationArbitraryAxis=[0 0 1]  FollAlignAxisA=+X  BaseAlignAxisA=+Y  FollAlignAxisB=+Y  BaseAlignAxisB=+Z  RotationSequenceAxes=FollowerAxes  RotationSequence=XYX  RotationSequenceAngles=[0 0 0]  RotationSequenceAnglesUnits=deg  RotationMatrix=[1 0 0; 0 1 0; 0 0 1]
  Sensor_1 : sm_lib/Body Elements/Spherical Solid  GraphicAmbientColor=[0.15 0.15 0.15 1.0]  BasedOnType=Density  CenterOfMass=[0 0 0]  CenterOfMassUnits=m  GraphicDiffuseColor=[0.9411765 0.9411765 0.9411765]  Density=1000  DensityUnits=kg/m^3  DoExposeReferenceFrame=on  GraphicEmissiveColor=[0.0 0.0 0.0 1.0]  ExportEntireGeometry=on  SerializedExposedGeometries=<ExposedGeometries><ExposedGeometry><RawGeometryId>entire</RawGeometryId><ExposedGeometryId>G</ExposedGeometryId></ExposedGeometry></ExposedGeometries>  SerializedFrames=<Frames/>  MarkerShape=Sphere  MarkerSize=10  GraphicType=FromGeometry  InertiaType=CalculateFromGeometry  Mass=1  MassUnits=kg  MomentsOfInertia=[1 1 1]  MomentsOfInertiaUnits=kg*m^2  GraphicOpacity=1.0  ProductsOfInertia=[0 0 0]  ProductsOfInertiaUnits=kg*m^2  GraphicShininess=75  GraphicSpecularColor=[0.5 0.5 0.5 1.0]  SphereRadius=0.1  SphereRadiusUnits=cm  GraphicVisPropType=SimpleVisualProperties
  Sensor_2 : sm_lib/Body Elements/Spherical Solid  GraphicAmbientColor=[0.15 0.15 0.15 1.0]  BasedOnType=Density  CenterOfMass=[0 0 0]  CenterOfMassUnits=m  GraphicDiffuseColor=[0.9411765 0.9411765 0.9411765]  Density=1000  DensityUnits=kg/m^3  DoExposeReferenceFrame=on  GraphicEmissiveColor=[0.0 0.0 0.0 1.0]  ExportEntireGeometry=on  SerializedExposedGeometries=<ExposedGeometries><ExposedGeometry><RawGeometryId>entire</RawGeometryId><ExposedGeometryId>G</ExposedGeometryId></ExposedGeometry></ExposedGeometries>  SerializedFrames=<Frames/>  MarkerShape=Sphere  MarkerSize=10  GraphicType=FromGeometry  InertiaType=CalculateFromGeometry  Mass=1  MassUnits=kg  MomentsOfInertia=[1 1 1]  MomentsOfInertiaUnits=kg*m^2  GraphicOpacity=1.0  ProductsOfInertia=[0 0 0]  ProductsOfInertiaUnits=kg*m^2  GraphicShininess=75  GraphicSpecularColor=[0.5 0.5 0.5 1.0]  SphereRadius=0.1  SphereRadiusUnits=cm  GraphicVisPropType=SimpleVisualProperties
  Simulink-PS Converter1 : nesl_utility/Simulink-PS Converter  PhysicalDomain=network_engine_domain  SubClassName=ps_input  LeftPortType=input  RightPortType=output  PseudoPeriodic=off  Frequencies=[]  NoiseDistribution=none  NoiseParameters=[]  Unit=1  AffineConversion=off  FilteringAndDerivatives=filter  SimscapeFilterOrder=2  InputFilterTimeConstant=0.001  UdotUserProvided=0
      settings: SourceProductBaseCode=PW,SS
  Simulink-PS Converter2 : nesl_utility/Simulink-PS Converter  PhysicalDomain=network_engine_domain  SubClassName=ps_input  LeftPortType=input  RightPortType=output  PseudoPeriodic=off  Frequencies=[]  NoiseDistribution=none  NoiseParameters=[]  Unit=1  AffineConversion=off  FilteringAndDerivatives=filter  SimscapeFilterOrder=2  InputFilterTimeConstant=0.001  UdotUserProvided=0
      settings: SourceProductBaseCode=PW,SS
  Simulink-PS Converter3 : nesl_utility/Simulink-PS Converter  PhysicalDomain=network_engine_domain  SubClassName=ps_input  LeftPortType=input  RightPortType=output  PseudoPeriodic=off  Frequencies=[]  NoiseDistribution=none  NoiseParameters=[]  Unit=1  AffineConversion=off  FilteringAndDerivatives=filter  SimscapeFilterOrder=2  InputFilterTimeConstant=0.001  UdotUserProvided=0
      settings: SourceProductBaseCode=PW,SS
  Transform Sensor : sm_lib/Frames and Transforms/Transform Sensor  MeasurementFrame=Follower  SenseAngle=off  SenseAxis=off  SenseAngle1=off  SenseAngle2=off  SenseAngle3=off  SenseQ=off  SenseR=off  SenseOmegaX=off  SenseOmegaY=off  SenseOmegaZ=off  SenseOmega1=off  SenseOmega2=off  SenseOmega3=off  SenseQDot=off  SenseRDot=off  SenseAlphaX=off  SenseAlphaY=off  SenseAlphaZ=off  SenseAlpha1=off  SenseAlpha2=off  SenseAlpha3=off  SenseQDDot=off  SenseRDDot=off  SenseX=off  SenseY=off  SenseZ=on  SenseRad=off  SenseAzim=off  SenseDist=off  SenseInc=off  SenseXDot=off  SenseYDot=off  SenseZDot=off  SenseRadDot=off  SenseAzimDot=off  SenseDistDot=off  SenseIncDot=off  SenseXDDot=off  SenseYDDot=off  SenseZDDot=off  SenseRadDDot=off  SenseAzimDDot=off  SenseDistDDot=off  SenseIncDDot=off
  Transform Sensor1 : sm_lib/Frames and Transforms/Transform Sensor  MeasurementFrame=Follower  SenseAngle=off  SenseAxis=off  SenseAngle1=off  SenseAngle2=off  SenseAngle3=off  SenseQ=off  SenseR=off  SenseOmegaX=off  SenseOmegaY=off  SenseOmegaZ=off  SenseOmega1=off  SenseOmega2=off  SenseOmega3=off  SenseQDot=off  SenseRDot=off  SenseAlphaX=off  SenseAlphaY=off  SenseAlphaZ=off  SenseAlpha1=off  SenseAlpha2=off  SenseAlpha3=off  SenseQDDot=off  SenseRDDot=off  SenseX=off  SenseY=off  SenseZ=on  SenseRad=off  SenseAzim=off  SenseDist=off  SenseInc=off  SenseXDot=off  SenseYDot=off  SenseZDot=off  SenseRadDot=off  SenseAzimDot=off  SenseDistDot=off  SenseIncDot=off  SenseXDDot=off  SenseYDDot=off  SenseZDDot=off  SenseRadDDot=off  SenseAzimDDot=off  SenseDistDDot=off  SenseIncDDot=off
  Conn2 : PMIOPort  Side=Left
  Conn3 : PMIOPort  Port=2  Side=Left
  Conn6 : PMIOPort  Port=3  Side=Left
  Conn4 : PMIOPort  Port=4  Side=Right
  Sensor_Dist_1 : Outport
  Sensor_Dist_2 : Outport  Port=2
  wires:
  PS-Simulink Converter/1 -> Sensor_Dist_1/1
  PS-Simulink Converter1/1 -> Sensor_Dist_2/1
  force1/1 -> Simulink-PS Converter2/1
  force2/1 -> Simulink-PS Converter1/1
  force3/1 -> Simulink-PS Converter3/1
  connections:
  Prismatic Joint/LConn1 -- Rigid Transform1/RConn1
  Brick Solid1/RConn1 -- Transform Sensor/LConn1 -- Rigid Transform1/LConn1 -- Transform Sensor1/LConn1 -- Rigid Transform/LConn1 -- Rigid Transform3/LConn1
  Transform Sensor/RConn1 -- Prismatic Joint/RConn1 -- Sensor_1/RConn1
  Conn3/RConn1 -- Middle_Sensor/LConn1
  Conn6/RConn1 -- Sensor_2/LConn1
  Prismatic Joint1/RConn1 -- Middle_Sensor/RConn1
  Prismatic Joint3/LConn1 -- Rigid Transform/RConn1
  Sensor_2/RConn1 -- Prismatic Joint3/RConn1 -- Transform Sensor1/RConn1
  Prismatic Joint1/LConn1 -- Rigid Transform3/RConn1
  PS-Simulink Converter/LConn1 -- Transform Sensor/RConn2
  Conn4/RConn1 -- Brick Solid1/LConn1
  Conn2/RConn1 -- Sensor_1/LConn1
  PS-Simulink Converter1/LConn1 -- Transform Sensor1/RConn2
  Prismatic Joint/LConn2 -- Simulink-PS Converter2/RConn1
  Prismatic Joint3/LConn2 -- Simulink-PS Converter1/RConn1
  Prismatic Joint1/LConn2 -- Simulink-PS Converter3/RConn1

== system FinalRobot/Snake/Verin ==
  Torq12 : Inport
  Torq11 : Inport  Port=2
  rot : Inport  Port=3
  Subsystem2 : Subsystem
      settings: PortSchema="{\"entries\":[{\"content\":{\"sides\":[{\"content\":{\"connectorIds\":[\"LConn1\"]},\"type\":\"ConnectorPlacement.EquallySpacedRectSide\",\"uuid\":\"928894c3-36c9-4b3f-8604-d5cfb900f216\"},{\"content\":{\"connectorIds\":[\"RConn1\"],\"side\":\"RIGHT\"},\"type\":\"ConnectorPlacement.EquallySpacedRectSide\",\"uuid\":\"1b973b4c-df80-49ba-8b37-588e61de75f2\"},{\"content\":{\"connectorIds\":[],\"side\":\"TOP\"},\"type\":\"ConnectorPlacement.EquallySpacedRectSide\",\"uuid\":\"c211ee3f-c814-40c3-a296-91b381758094\"},{\"content\":{\"connectorIds\":[\"RConn2\",\"In1\"],\"side\":\"BOTTOM\"},\"type\":\"ConnectorPlacement.EquallySpacedRectSide\",\"uuid\":\"65b28e6d-8020-404b-a81e-d6d35fec57aa\"}]},\"type\":\"ConnectorPlacement.EquallySpacedConnector\",\"uuid\":\"69690137-dd1f-43cb-9e25-3381f1b9516d\"}],\"packageUris\":[\"http://schema.mathworks.com/mf0/Connector/R2020b\"],\"version\":\"1.0\"}"
      mask Display: image('$imagefile'); % Use "Edit Image" on toolstrip to change.
  Subsystem3 : Subsystem
      settings: PortSchema="{\"entries\":[{\"content\":{\"sides\":[{\"content\":{\"connectorIds\":[\"LConn1\"]},\"type\":\"ConnectorPlacement.EquallySpacedRectSide\",\"uuid\":\"fb7ca892-623b-4289-934f-aee105276814\"},{\"content\":{\"connectorIds\":[\"RConn1\"],\"side\":\"RIGHT\"},\"type\":\"ConnectorPlacement.EquallySpacedRectSide\",\"uuid\":\"0daf8b48-229f-46bb-9482-184447c743c5\"},{\"content\":{\"connectorIds\":[\"In1\",\"In2\",\"Out1\",\"Out2\"],\"side\":\"TOP\"},\"type\":\"ConnectorPlacement.EquallySpacedRectSide\",\"uuid\":\"c258a386-6c23-4ebb-b6ca-e534711f920f\"},{\"content\":{\"connectorIds\":[\"RConn2\",\"RConn3\",\"RConn4\",\"RConn5\"],\"side\":\"BOTTOM\"},\"type\":\"ConnectorPlacement.EquallySpacedRectSide\",\"uuid\":\"3e83ec0e-900d-4924-8cc6-19cde9453293\"}]},\"type\":\"ConnectorPlacement.EquallySpacedConnector\",\"uuid\":\"dfcdae3d-d414-45a1-b62e-1dc7d14d079d\"}],\"packageUris\":[\"http://schema.mathworks.com/mf0/Connector/R2020b\"],\"version\":\"1.0\"}"
      mask Display: image('$imagefile'); % Use "Edit Image" on toolstrip to change.
  Conn1 : PMIOPort  Side=Left
  Conn3 : PMIOPort  Port=2  Side=Right
  Amor : PMIOPort  Port=3  Side=Right
  H_Verin : PMIOPort  Port=4  Side=Right
  B_Verin : PMIOPort  Port=5  Side=Right
  Ref1 : PMIOPort  Port=6  Side=Right
  azm1 : Outport
  v1 : Outport  Port=2
  wires:
  Torq12/1 -> Subsystem3/1(input0)
  Torq11/1 -> Subsystem3/2(input1)
  Subsystem3/1(azm1) -> azm1/1
  rot/1 -> Subsystem2/1(input0)
  Subsystem3/2(v1) -> v1/1
  connections:
  Subsystem3/RConn2 -- Amor/RConn1
  Conn1/RConn1 -- Subsystem3/LConn1
  Subsystem3/RConn3 -- H_Verin/RConn1
  Subsystem3/RConn4 -- B_Verin/RConn1
  Subsystem3/RConn1 -- Subsystem2/LConn1
  Ref1/RConn1 -- Subsystem3/RConn5 -- Subsystem2/RConn2
  Subsystem2/RConn1 -- Conn3/RConn1

== system FinalRobot/Snake/Verin1 ==
  Torq22 : Inport
  Torq21 : Inport  Port=2
  Camera : sm_lib/Body Elements/Spherical Solid  GraphicAmbientColor=[0.15 0.15 0.15 1.0]  BasedOnType=Density  CenterOfMass=[0 0 0]  CenterOfMassUnits=m  GraphicDiffuseColor=[0.9411765 0.9411765 0.9411765]  Density=10  DensityUnits=kg/m^3  DoExposeReferenceFrame=on  GraphicEmissiveColor=[0.0 0.0 0.0 1.0]  ExportEntireGeometry=off  SerializedExposedGeometries=<ExposedGeometries/>  SerializedFrames=<Frames/>  MarkerShape=Sphere  MarkerSize=10  GraphicType=FromGeometry  InertiaType=CalculateFromGeometry  Mass=1  MassUnits=kg  MomentsOfInertia=[1 1 1]  MomentsOfInertiaUnits=kg*m^2  GraphicOpacity=0  ProductsOfInertia=[0 0 0]  ProductsOfInertiaUnits=kg*m^2  GraphicShininess=75  GraphicSpecularColor=[0.5 0.5 0.5 1.0]  SphereRadius=0.1  SphereRadiusUnits=cm  GraphicVisPropType=SimpleVisualProperties
  Revolute Joint1 : sm_lib/Joints/Revolute Joint  JointMode=Normal  SenseConstraintForce=off  SenseConstraintForceX=off  SenseConstraintForceY=off  SenseConstraintForceZ=off  SenseConstraintTorque=off  SenseConstraintTorqueX=off  SenseConstraintTorqueY=off  SenseConstraintTorqueZ=off  SenseTotalForce=off  SenseTotalForceX=off  SenseTotalForceY=off  SenseTotalForceZ=off  SenseTotalTorque=off  SenseTotalTorqueX=off  SenseTotalTorqueY=off  SenseTotalTorqueZ=off  CompositeWrenchDir=FollowerOnBase  CompositeWrenchFrame=BaseFrame  EquilibriumPosition=0  EquilibriumPositionUnits=deg  SpringStiffness=Stiffness_Spine  SpringStiffnessUnits=N*m/deg  DampingCoefficient=Damping_Spine  DampingCoefficientUnits=N*m/(deg/s)  TorqueActuationMode=NoTorque  MotionActuationMode=ComputedMotion  SensePosition=off  SenseVelocity=off  SenseAcceleration=off  SenseTorqueForce=off  SenseLowerLimitTorqueForce=off  SenseUpperLimitTorqueForce=off  LowerLimitSpecify=off  LowerLimitBound=-90  LowerLimitBoundUnits=deg  LowerLimitStiffness=1e4  LowerLimitStiffnessUnits=N*m/deg  LowerLimitDamping=10  LowerLimitDampingUnits=N*m/(deg/s)  LowerLimitTransitionRegionWidth=0.1  LowerLimitTransitionRegionWidthUnits=deg  UpperLimitSpecify=off  UpperLimitBound=90  UpperLimitBoundUnits=deg  UpperLimitStiffness=1e4  UpperLimitStiffnessUnits=N*m/deg  UpperLimitDamping=10  UpperLimitDampingUnits=N*m/(deg/s)  UpperLimitTransitionRegionWidth=0.1  UpperLimitTransitionRegionWidthUnits=deg  PositionTargetSpecify=off  PositionTargetPriority=High  PositionTargetValue=0  PositionTargetValueUnits=deg  VelocityTargetSpecify=off  VelocityTargetPriority=High  VelocityTargetValue=0  VelocityTargetValueUnits=deg/s
  Rigid Transform4 : sm_lib/Frames and Transforms/Rigid Transform  TranslationMethod=Cartesian  TranslationStandardOffset=-10  TranslationLengthUnit=m  TranslationStandardAxis=+Z  TranslationCartesianOffset=[0 -0.1 0.1]  TranslationROffset=0  TranslationROffsetUnits=m  TranslationZOffset=0  TranslationZOffsetUnits=m  TranslationThetaOffset=0  TranslationThetaOffsetUnits=deg  RotationMethod=StandardAxis  RotationAngleUnits=deg  RotationStandardAxis=+Z  RotationAngle=-10  RotationArbitraryAxis=[0 0 1]  FollAlignAxisA=+X  BaseAlignAxisA=+Y  FollAlignAxisB=+Y  BaseAlignAxisB=+Z  RotationSequenceAxes=FollowerAxes  RotationSequence=XYX  RotationSequenceAngles=[-45 45 0]  RotationSequenceAnglesUnits=deg  RotationMatrix=[1 0 0; 0 1 0; 0 0 1]
  Subsystem1 : Subsystem
      mask Display: image('C:\Users\MINGO Monique\Pictures\MatLab images\MatLab_img3.PNG'); % Use "Edit Image" on toolstrip to change.
  Subsystem3 : Subsystem
      settings: PortSchema="{\"entries\":[{\"content\":{\"sides\":[{\"content\":{\"connectorIds\":[\"LConn1\"]},\"type\":\"ConnectorPlacement.EquallySpacedRectSide\",\"uuid\":\"fb7ca892-623b-4289-934f-aee105276814\"},{\"content\":{\"connectorIds\":[\"RConn1\"],\"side\":\"RIGHT\"},\"type\":\"ConnectorPlacement.EquallySpacedRectSide\",\"uuid\":\"0daf8b48-229f-46bb-9482-184447c743c5\"},{\"content\":{\"connectorIds\":[\"In1\",\"In2\",\"Out1\",\"Out2\"],\"side\":\"TOP\"},\"type\":\"ConnectorPlacement.EquallySpacedRectSide\",\"uuid\":\"c258a386-6c23-4ebb-b6ca-e534711f920f\"},{\"content\":{\"connectorIds\":[\"RConn2\",\"RConn3\",\"RConn4\",\"RConn5\"],\"side\":\"BOTTOM\"},\"type\":\"ConnectorPlacement.EquallySpacedRectSide\",\"uuid\":\"3e83ec0e-900d-4924-8cc6-19cde9453293\"}]},\"type\":\"ConnectorPlacement.EquallySpacedConnector\",\"uuid\":\"dfcdae3d-d414-45a1-b62e-1dc7d14d079d\"}],\"packageUris\":[\"http://schema.mathworks.com/mf0/Connector/R2020b\"],\"version\":\"1.0\"}"
      mask Display: image('$imagefile'); % Use "Edit Image" on toolstrip to change.
  Subsystem5 : Subsystem
      mask Display: image('C:\Users\MINGO Monique\Pictures\MatLab images\MatLab_img2.PNG'); % Use "Edit Image" on toolstrip to change.
  Conn1 : PMIOPort  Side=Left
  Conn3 : PMIOPort  Port=2  Side=Right
  Amor1 : PMIOPort  Port=3  Side=Right
  H_Verin : PMIOPort  Port=4  Side=Right
  B_Verin : PMIOPort  Port=5  Side=Right
  Ref1 : PMIOPort  Port=6  Side=Right
  Ref2 : PMIOPort  Port=7  Side=Right
  azm2 : Outport
  wz2 : Outport  Port=2
  wires:
  Torq22/1 -> Subsystem3/1(input0)
  Torq21/1 -> Subsystem3/2(input1)
  Subsystem3/1(azm2) -> azm2/1
  Subsystem3/2(wz2) -> wz2/1
  connections:
  Conn1/RConn1 -- Subsystem3/LConn1
  Amor1/RConn1 -- Subsystem3/RConn2
  H_Verin/RConn1 -- Subsystem3/RConn3
  B_Verin/RConn1 -- Subsystem3/RConn4
  Subsystem5/RConn1 -- Rigid Transform4/LConn1 -- Conn3/RConn1
  Ref1/RConn1 -- Subsystem3/RConn5
  Ref2/RConn1 -- Revolute Joint1/RConn1 -- Subsystem1/RConn1
  Subsystem1/LConn1 -- Subsystem3/RConn1
  Revolute Joint1/LConn1 -- Subsystem5/LConn1
  Camera/RConn1 -- Rigid Transform4/RConn1
